simulink model "SeperatelyExcited"  (R2019a)
settings: Solver=VariableStepAuto  StartTime=0.0  StopTime=10.0  RelTol=1e-3
InitFcn:
  | run MotorParameter_Initialize
values from neighbouring files (symbols this model uses):
  Bm = 0    [MotorParameter_Initialize.m]
  J = 0.02    [MotorParameter_Initialize.m]
  Laa = 60e-3    (= 0.06)    [MotorParameter_Initialize.m]
  Laf = 3.8    [MotorParameter_Initialize.m]
  Lff = 50    [MotorParameter_Initialize.m]
  Ra = 3.6    [MotorParameter_Initialize.m]
  Rf = 450    [MotorParameter_Initialize.m]
settings Model: Creator=visha  LastModifiedBy=visha

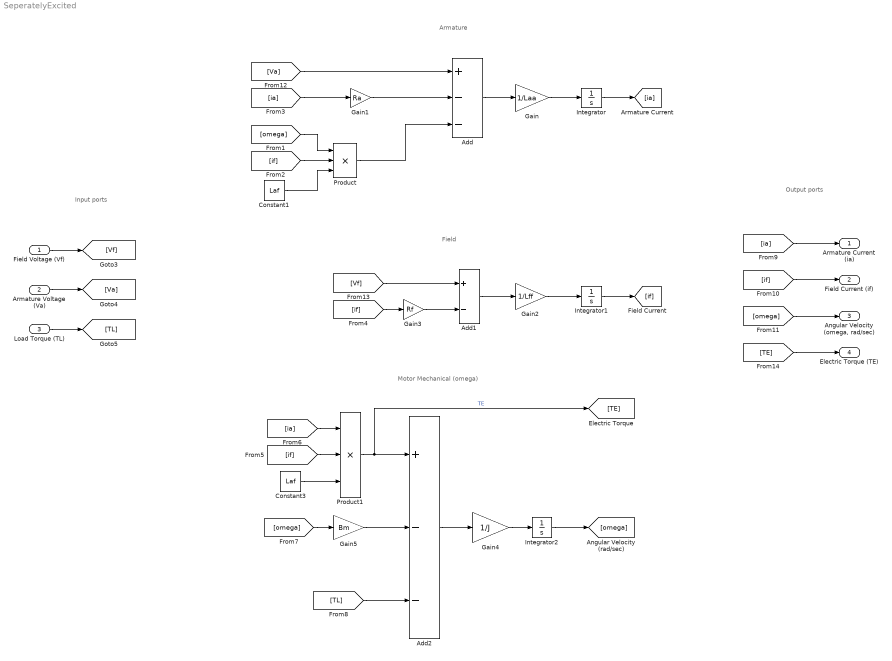
== system SeperatelyExcited ==
  note: Field
  note: Armature
  note: Motor Mechanical (omega)
  note: Output ports
  note: Input ports
  Field Voltage (Vf) : Inport
  Armature Voltage (Va) : Inport  Port=2
  Load Torque (TL) : Inport  Port=3
  Add : Sum  Inputs=+--
  Add1 : Sum  Inputs=+-
  Add2 : Sum  Inputs=+--
  Constant1 : Constant  Value=Laf
  Constant3 : Constant  Value=Laf
  Gain : Gain  Gain=1/Laa
  Gain1 : Gain  Gain=Ra
  Gain2 : Gain  Gain=1/Lff
  Gain3 : Gain  Gain=Rf
  Gain4 : Gain  Gain=1/J
  Gain5 : Gain  Gain=Bm
  Integrator : Integrator
  Integrator1 : Integrator
  Integrator2 : Integrator
  Product : Product  Inputs=3
  Product1 : Product  Inputs=3
  Armature Current (ia) : Outport
  Field Current (if) : Outport  Port=2
  "Angular Velocity (omega, rad/sec)" : Outport  Port=3
  Electric Torque (TE) : Outport  Port=4
  wires:
  Gain/1 -> Integrator/1
  Add/1 -> Gain/1
  Integrator/1 -> [ia]
  [ia] -> Gain1/1
  Gain1/1 -> Add/2
  [if] -> Product/2
  [omega] -> Product/1
  Constant1/1 -> Product/3
  Product/1 -> Add/3
  Integrator1/1 -> [if]
  Gain2/1 -> Integrator1/1
  Gain3/1 -> Add1/2
  [Vf] -> Add1/1
  [if] -> Gain3/1
  Add1/1 -> Gain2/1
  [ia] -> Product1/1
  [if] -> Product1/2
  Constant3/1 -> Product1/3
  Add2/1 -> Gain4/1
  Product1/1 -> [TE], Add2/1  "TE"
  Gain4/1 -> Integrator2/1
  Integrator2/1 -> [omega]
  Gain5/1 -> Add2/2
  [omega] -> Gain5/1
  [TL] -> Add2/3
  [ia] -> Armature Current (ia)/1
  [if] -> Field Current (if)/1
  [omega] -> "Angular Velocity (omega, rad/sec)"/1
  [Va] -> Add/1
  Field Voltage (Vf)/1 -> [Vf]
  Armature Voltage (Va)/1 -> [Va]
  Load Torque (TL)/1 -> [TL]
  [TE] -> Electric Torque (TE)/1
